simulink model "hw2d"  (R2017a)
settings: Solver=VariableStepAuto  StartTime=0.0  StopTime=10.0  RelTol=1e-3
settings Model: Creator=Soutrik  LastModifiedBy=Soutrik

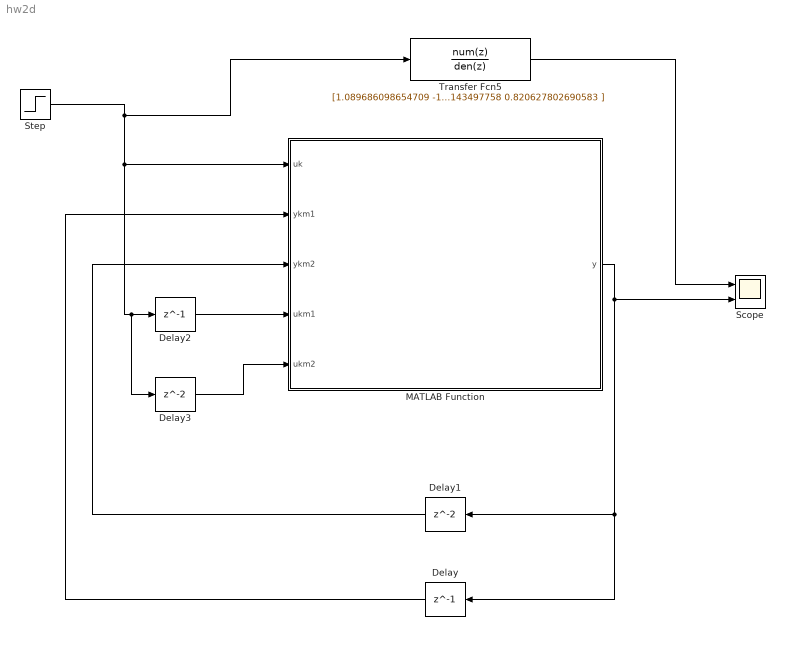
== system hw2d ==
  Delay : Delay  DelayLength=1  InitialCondition=0
  Delay1 : Delay  InitialCondition=0
  Delay2 : Delay  DelayLength=1  InitialCondition=0
  Delay3 : Delay  InitialCondition=0
  MATLAB Function : MATLAB Function  TreatAsAtomicUnit=on
  Scope : Scope  NumInputPorts=2
  Step : Step  SampleTime=0.1  mask(DiscretizedSource){}
      mask init:
      | %tustin
  Transfer Fcn5 : DiscreteTransferFcn  Numerator=[1.089686098654709 -1.766816143497758 0.730941704035875 ]  Denominator=[1.000000000000000 -1.766816143497758 0.820627802690583 ]  SampleTime=0.10000000000000001
  wires:
  MATLAB Function/1(y) -> Scope/2, Delay1/1, Delay/1
  Delay/1 -> MATLAB Function/2(ykm1)
  Delay1/1 -> MATLAB Function/3(ykm2)
  Step/1 -> Transfer Fcn5/1, MATLAB Function/1(uk), Delay3/1, Delay2/1
  Delay2/1 -> MATLAB Function/4(ukm1)
  Delay3/1 -> MATLAB Function/5(ukm2)
  Transfer Fcn5/1 -> Scope/1

== matlab function hw2d/MATLAB Function ==
  data: uk input; y output; ykm1 input; ykm2 input; ukm1 input; ukm2 input
function y = fcn(uk,ykm1,ykm2,ukm1,ukm2)
y=1.767*ykm1-0.8206*ykm2+1.09*uk-1.767*ukm1+0.7309*ukm2;
